simulink model "PID_MassSDModel"  (R2025a)
settings: Solver=VariableStepAuto  StartTime=0.0  StopTime=10.0  RelTol=1e-3
undefined symbols (not defined in the file): b, F, k, Kd, Ki, Kp, M
settings Model: Creator=Pablo  LastModifiedBy=Pablo

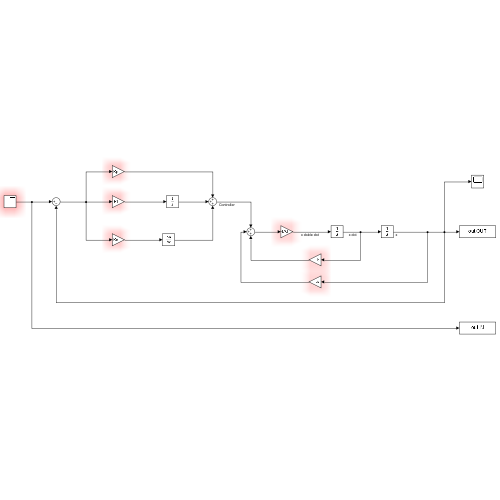
[thumbnail: Simulink's stored preview of the top-level diagram]
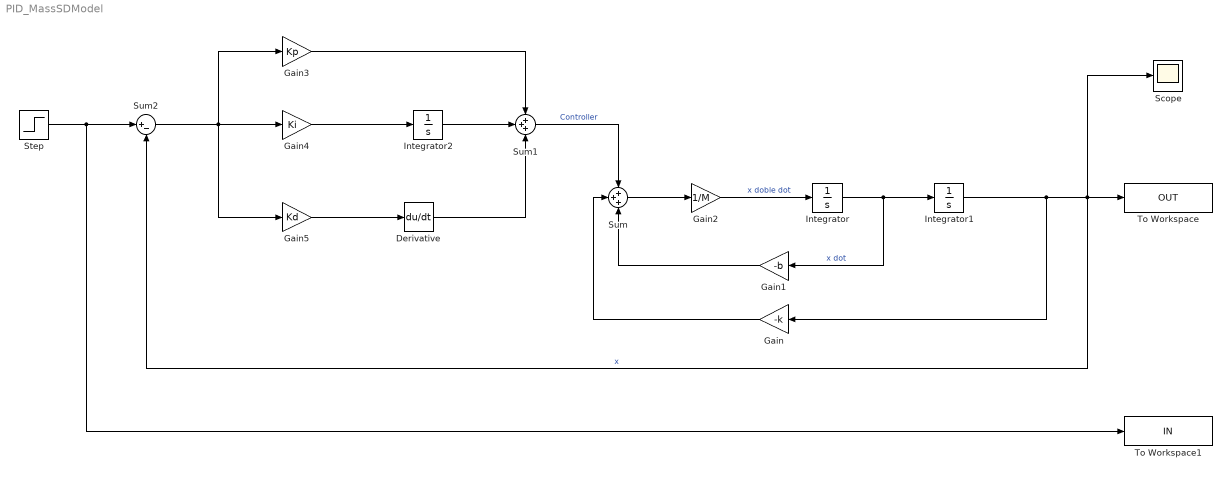
== system PID_MassSDModel ==
  Derivative : Derivative
  Gain : Gain  Gain=-k
  Gain1 : Gain  Gain=-b
  Gain2 : Gain  Gain=1/M
  Gain3 : Gain  Gain=Kp
  Gain4 : Gain  Gain=Ki
  Gain5 : Gain  Gain=Kd
  Integrator : Integrator
  Integrator1 : Integrator
  Integrator2 : Integrator
  Scope : Scope
  Step : Step  Time=F  After=F  SampleTime=0
  Sum : Sum  Inputs=+++
  Sum1 : Sum  Inputs=+++
  Sum2 : Sum  Inputs=|+-
  To Workspace : ToWorkspace  VariableName=OUT  SaveFormat=Timeseries  SampleTime=-1
  To Workspace1 : ToWorkspace  VariableName=IN  SaveFormat=Timeseries  SampleTime=-1
  wires:
  Integrator/1 -> Gain1/1, Integrator1/1  "x dot"
  Integrator1/1 -> Scope/1, To Workspace/1, Sum2/2, Gain/1  "x"
  Gain2/1 -> Integrator/1  "x doble dot"
  Gain1/1 -> Sum/3
  Gain/1 -> Sum/2
  Sum/1 -> Gain2/1
  Gain4/1 -> Integrator2/1
  Gain3/1 -> Sum1/1
  Derivative/1 -> Sum1/3
  Integrator2/1 -> Sum1/2
  Gain5/1 -> Derivative/1
  Sum1/1 -> Sum/1  "Controller"
  Step/1 -> To Workspace1/1, Sum2/1
  Sum2/1 -> Gain5/1, Gain3/1, Gain4/1
